simulink model "simulink_template_2_3"  (R2024b)
settings: Solver=VariableStepAuto  StartTime=0.0  StopTime=total_time  RelTol=1e-3
values from neighbouring files (symbols this model uses):
  mode = 1    [MAIN.m]
  qf = [1,1,pi/3]'    [MAIN.m]
  qi = [0,0,-pi/3]'    [MAIN.m]
  total_time = 10    [MAIN.m]
settings Model: Creator=alber  LastModifiedBy=cosmi
settings RTWCC: GPUComputeCapability=3.5

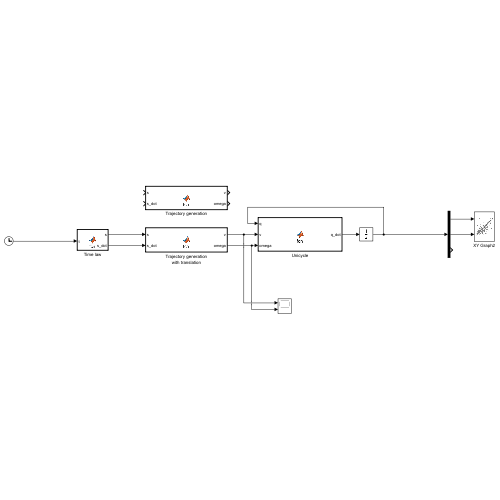
[thumbnail: Simulink's stored preview of the top-level diagram]
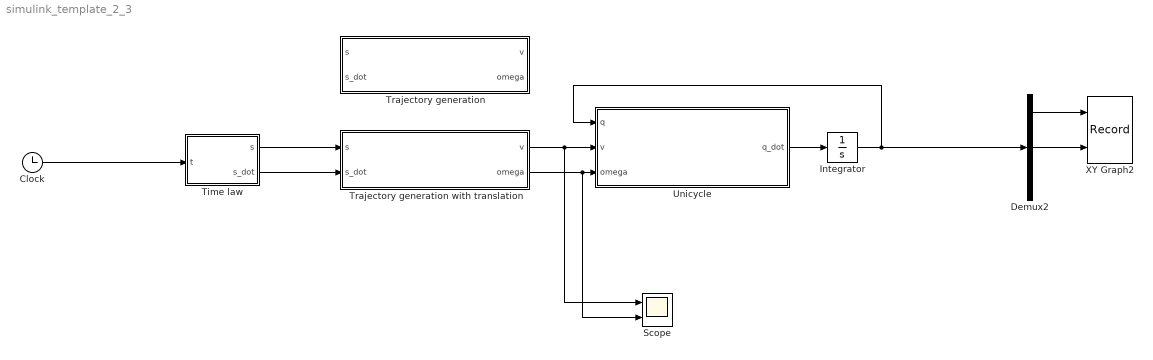
== system simulink_template_2_3 ==
  Clock : Clock
  Demux2 : Demux  Outputs=3
  Integrator : Integrator  InitialCondition=qi
  Scope : Scope  NumInputPorts=2
  Time law : MATLAB Function  TreatAsAtomicUnit=on
  Trajectory generation : MATLAB Function  TreatAsAtomicUnit=on
  Trajectory generation with translation : MATLAB Function  TreatAsAtomicUnit=on
  Unicycle : MATLAB Function  TreatAsAtomicUnit=on
  XY Graph2 : Record  FileSettingsInternal="{\"entries\":[{\"content\":{\"excelSettings\":{\"content\":{},\"type\":\"Streamout.ExcelSettings\"}},\"type\":\"Streamout.FileSettingStorage\",\"uuid\":\"\"}],\"packageUris\":[\"http:\\/\\/schema.mathworks.com\\/mf0\\/streamout_blocks\\/R2020a\"],\"version\":\"1.0\"}"  Layout=[1 1]  SignalsInternal="{\"entries\":[{\"content\":{\"signals\":[{\"content\":{\"blockPath\":[],\"dimensions\":[1,1],\"domain\":\"\",\"lineColor\":\"#a2142f\",\"plots\":[ 1 ],\"port\":1,\"signalID\":1,\"signalName\":\"Demux2:1\"},\"type\":\"RecordBlkView.Signal\",\"uuid\":\"\"},{\"content\":{\"blockPath\":[],\"dimensions\":[1,1],\"domain\":\"\",\"lineColor\":\"#139fff\",\"plots\":[ 1 ],\"port\":2,\"signalID\":2,\"signalName\":\"Demux2:2\"},\"type\":\"RecordBlkView.Signal\",\"uuid\":\"\"}]},\"type\":\"RecordBlkView.InputSignals\",\"uuid\":\"\"}],\"packageUris\":[\"http:\\/\\/schema.mathworks.com\\/mf0\\/streamout_blocks\\/R2020a\"],\"version\":\"1.0\"}"  VisualizationBindings="{\"xyplotplugin\":{\"info\":[{\"series\":[{\"bindingParametersList\":[{\"parameter\":\"X-Axis\",\"signalID\":1,\"signalName\":\"Demux2:1\"},{\"parameter\":\"Y-Axis\",\"signalID\":2,\"signalName\":\"Demux2:2\"}],\"seriesID\":0}],\"subplotID\":1}]}}"  CompatibilityTag=XY
  wires:
  Time law/1(s) -> Trajectory generation with translation/1(s)
  Time law/2(s_dot) -> Trajectory generation with translation/2(s_dot)
  Trajectory generation with translation/1(v) -> Unicycle/2(v), Scope/1
  Trajectory generation with translation/2(omega) -> Scope/2, Unicycle/3(omega)
  Unicycle/1(q_dot) -> Integrator/1
  Integrator/1 -> Demux2/1, Unicycle/1(q)
  Demux2/2 -> XY Graph2/2
  Demux2/1 -> XY Graph2/1
  Clock/1 -> Time law/1(t)

== matlab function simulink_template_2_3/Trajectory generation ==
  data: v output; s input; s_dot input; omega output; qi parameter; qf parameter
function [v , omega] = fcn(s, s_dot, qi, qf)

zi = [qi(3);
    qi(1)*cos(qi(3)) + qi(2)*sin(qi(3));
    qi(1)*sin(qi(3)) - qi(2)*cos(qi(3));
    ];

zf = [qf(3);
    qf(1)*cos(qf(3)) + qf(2)*sin(qf(3));
    qf(1)*sin(qf(3)) - qf(2)*cos(qf(3));
    ];

if(zi(1)==zf(1))
    zf(1) = zi(1) + (2*pi);
end

a = [zf(1),zi(1)];
b = [zf(3) , zi(3) , zf(2)*(zf(1)-zi(1)) - 3*zf(3) , zi(2)*(zf(1)-zi(1)) + 3*zi(3)];


z1 = a(1)*s - a(2)*(s-1);
z1_dot = a(1) - a(2);

z3 = b(1)*(s^3) - b(2)*((s-1)^3) + b(3)*(s-1)*(s^2) + b(4)*s*((s-1)^2);
z3_dot = b(1)*(s^2)*3 - b(2)*((s-1)^2)*3 + b(3)*(s^2 + 2*(s-1)*s) + b(4)*((s-1)^2 + s*2*(s-1));
z3_ddot = b(1)*(s)*6 - b(2)*((s-1))*6 + b(3)*(s*2 + 2*(s*2-1)) + b(4)*((s-1)*2 + 2*(s*2-1));

z2 = z3_dot/z1_dot;
z2_dot = (z3_ddot)/((a(1) - a(2)));


omega = (zf(1)-zi(1))*s_dot;
%v = ((zf(1)-zi(1))*z3+(z3_ddot/z1_dot))*s_dot;


v = ((zf(1)-zi(1))*z3+z2_dot)*s_dot;

== matlab function simulink_template_2_3/Trajectory generation with translation ==
  data: v output; s input; s_dot input; omega output; qi parameter; qf parameter
function [v , omega] = fcn(s, s_dot, qi, qf)

zi = [qi(3);
    (qi(1)-qi(1))*cos(qi(3)) + (qi(2)-qi(2))*sin(qi(3));
    (qi(1)-qi(1))*sin(qi(3)) - (qi(2)-qi(2))*cos(qi(3));
    ];

zf = [qf(3);
    -(qi(1) - qf(1))*cos(qf(3)) - (qi(2) - qf(2))*sin(qf(3));
    -(qi(1) - qf(1))*sin(qf(3)) + (qi(2) - qf(2))*cos(qf(3))
    ];


if(zi(1)==zf(1))
    zf(1) = zi(1) + (2*pi);
end

a = [zf(1),zi(1)];
b = [zf(3) , zi(3) , zf(2)*(zf(1)-zi(1)) - 3*zf(3) , zi(2)*(zf(1)-zi(1)) + 3*zi(3)];


z1 = a(1)*s - a(2)*(s-1);
z1_dot = a(1) - a(2);

z3 = b(1)*(s^3) - b(2)*((s-1)^3) + b(3)*(s-1)*(s^2) + b(4)*s*((s-1)^2);
z3_dot = b(1)*(s^2)*3 - b(2)*((s-1)^2)*3 + b(3)*(s^2 + 2*(s-1)*s) + b(4)*((s-1)^2 + s*2*(s-1));
z3_ddot = b(1)*(s)*6 - b(2)*((s-1))*6 + b(3)*(s*2 + 2*(s*2-1)) + b(4)*((s-1)*2 + 2*(s*2-1));

z2 = z3_dot/z1_dot;
z2_dot = (z3_ddot)/((a(1) - a(2)));


omega = (zf(1)-zi(1))*s_dot;
%v = ((zf(1)-zi(1))*z3+(z3_ddot/z1_dot))*s_dot;


v = ((zf(1)-zi(1))*z3+z2_dot)*s_dot;

== matlab function simulink_template_2_3/Unicycle ==
  data: q_dot output; q input; v input; omega input
function q_dot = fcn(q, v, omega)
q_dot = [v*cos(q(3));v*sin(q(3));omega];

== matlab function simulink_template_2_3/Time law ==
  data: t input; s output; s_dot output; total_time parameter; mode parameter
function [s, s_dot] = fcn(t,total_time,mode)
s=0;
s_dot=0;
if mode==1%if mode =1 costasnt time law else trapezoidal
    s_dot = 1/total_time;
    s=t/total_time;
else
    Ta=0.1*total_time;% acceleration/dec time 10% of total
    Tc=total_time-2*Ta;%time of costant time

    Vc=1/(Ta+Tc);% velocità costante
    a=Vc/Ta;% acceleration
    switch 1 %formula on the slide
        case t<Ta
            s_dot=a*t;
            s=(a*(t^2))/2;

        case (t>=Ta)&&(t<(Tc+Ta))
            s_dot=Vc;
            s=(a*(Ta^2))/2+Vc*(t-Ta);

        case (t>=(Tc+Ta))&&(t<(Tc+2*Ta))
            s_dot=Vc-a*(t-Ta-Tc);
            s=(a*(Ta^2))/2+Vc*Tc+Vc*(t-Ta-Tc)-a*(t-Ta-Tc)^2/2;

        case t>=(Tc+2*Ta)
            s_dot=0;
            s=1;
    end

end
